simulink model "statefeebback_poleplacement"  (R2018b)
settings: Solver=VariableStepAuto  StartTime=0.0  StopTime=30  RelTol=1e-3
settings Model: Creator=Alireza  LastModifiedBy=Alireza

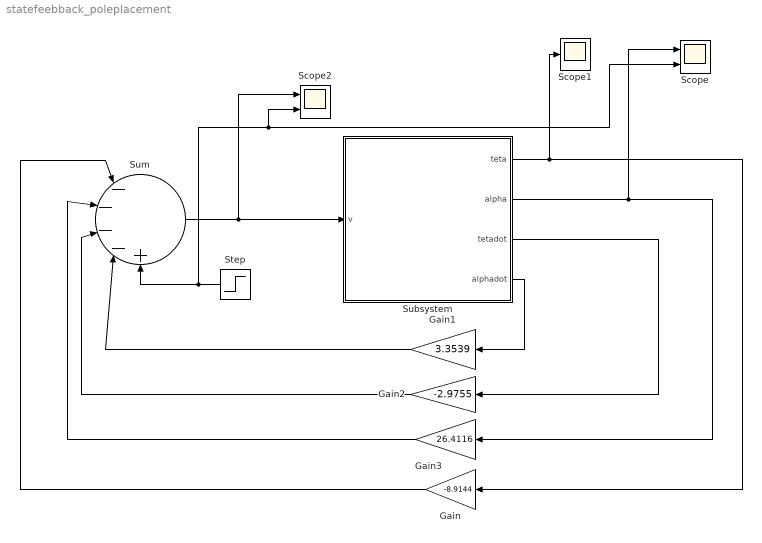
== system statefeebback_poleplacement ==
  Gain : Gain  Gain=-8.9144
  Gain1 : Gain  Gain=3.3539
  Gain2 : Gain  Gain=-2.9755
  Gain3 : Gain  Gain=26.4116
  Scope : Scope  NumInputPorts=2
  Scope1 : Scope
  Scope2 : Scope  NumInputPorts=2
  Step : Step  Time=3  Before=1  After=0  SampleTime=0
  Subsystem : Subsystem
  Sum : Sum  Inputs=|----+
  wires:
  Sum/1 -> Scope2/1, Subsystem/1(v)
  Subsystem/1(teta) -> Scope1/1, Gain/1
  Subsystem/2(alpha) -> Scope/1, Gain3/1
  Subsystem/3(tetadot) -> Gain2/1
  Subsystem/4(alphadot) -> Gain1/1
  Gain1/1 -> Sum/4
  Gain2/1 -> Sum/3
  Gain3/1 -> Sum/2
  Gain/1 -> Sum/1
  Step/1 -> Scope2/2, Scope/2, Sum/5

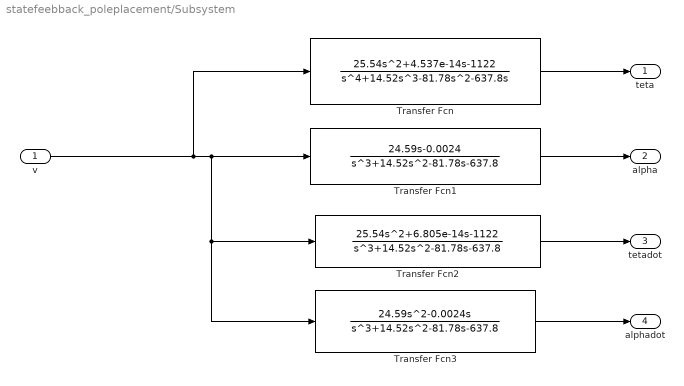
== system statefeebback_poleplacement/Subsystem ==
  v : Inport
  Transfer Fcn : TransferFcn  Numerator=[25.54 4.537e-14 -1122]  Denominator=[1 14.52 -81.78 -637.8 0]
  Transfer Fcn1 : TransferFcn  Numerator=[24.59 -0.0024]  Denominator=[1 14.52 -81.78 -637.8]
  Transfer Fcn2 : TransferFcn  Numerator=[25.54 6.805e-14 -1122]  Denominator=[1 14.52 -81.78 -637.8]
  Transfer Fcn3 : TransferFcn  Numerator=[24.59 -0.0024 0]  Denominator=[1 14.52 -81.78 -637.8]
  teta : Outport
  alpha : Outport  Port=2
  tetadot : Outport  Port=3
  alphadot : Outport  Port=4
  wires:
  v/1 -> Transfer Fcn1/1, Transfer Fcn3/1, Transfer Fcn2/1, Transfer Fcn/1
  Transfer Fcn/1 -> teta/1
  Transfer Fcn3/1 -> alphadot/1
  Transfer Fcn1/1 -> alpha/1
  Transfer Fcn2/1 -> tetadot/1
